simulink model "servomotor_posicao_EKF_Com_Ruido_Posicao"  (R2024b)
settings: Solver=FixedStepAuto  StartTime=0.0  StopTime=tf  FixedStep=1e-6  RelTol=1e-3
values from neighbouring files (symbols this model uses):
  controlador =     [controlador.mat]    (also in projetarControladorPosicaoOtimizacao.m = projetarControladorPosicaoAnalitico(requisitos, planta))
  planta =     [controlador.mat]    (also in kalman.m = obterPlantaServoPosicao())
undefined symbols (not defined in the file or in its folder): Continuous, Time
libraries: ctrlSharedLib x1
settings Model: Creator=mmaximo  LastModifiedBy=phdfo
settings SolverCC: AlgebraicLoopSolver=TrustRegion
settings DebuggingCC: UnconnectedInputMsg=warning  UnconnectedOutputMsg=warning  UnconnectedLineMsg=warning
settings ModelReferenceCC: EnableRefExpFcnMdlSchedulingChecks=on
settings RTWCC: GPUComputeCapability=3.5

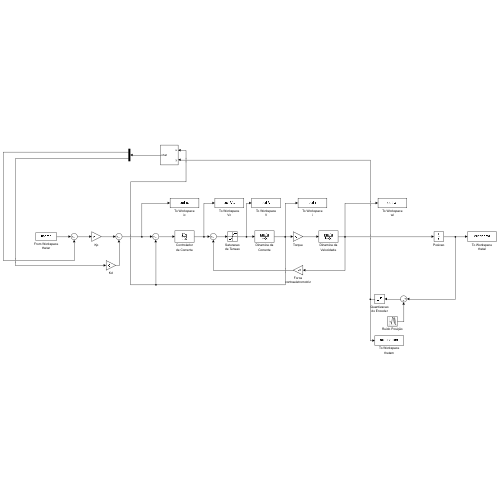
[thumbnail: Simulink's stored preview of the top-level diagram]
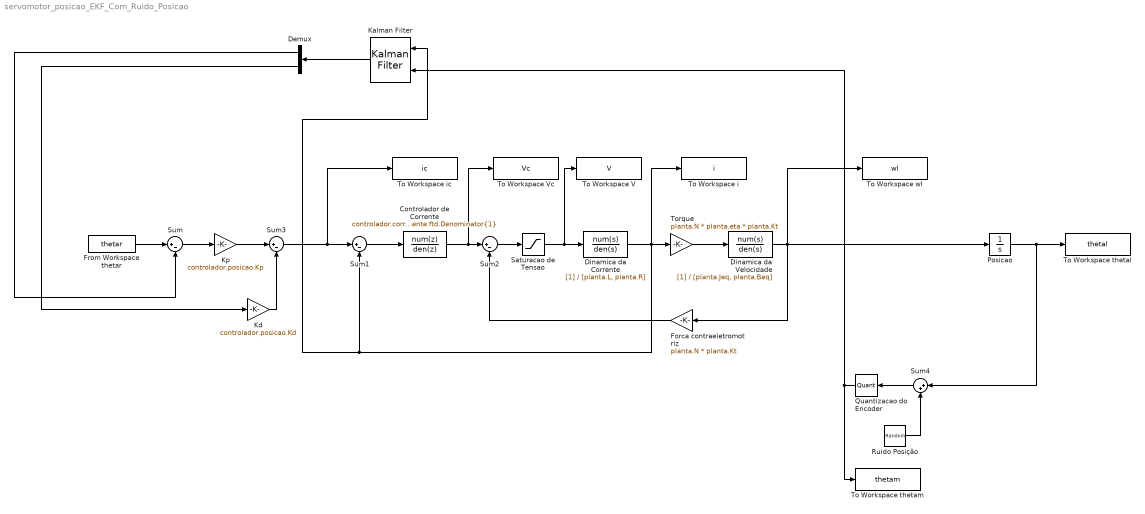
== system servomotor_posicao_EKF_Com_Ruido_Posicao ==
  Controlador de Corrente : DiscreteTransferFcn  Numerator=controlador.corrente.ftd.Numerator{1}  Denominator=controlador.corrente.ftd.Denominator{1}  SampleTime=controlador.corrente.T
  Demux : Demux  Outputs=2
  Dinamica da Corrente : TransferFcn  Denominator=[planta.L, planta.R]
  Dinamica da Velocidade : TransferFcn  Denominator=[planta.Jeq, planta.Beq]
  Forca contraeletromotriz : Gain  Gain=planta.N * planta.Kt
  From Workspace thetar : FromWorkspace  VariableName=thetar
  Kalman Filter : ctrlSharedLib/Kalman Filter  TimeDomain=Continuous-Time  UseCurrentEstimator=on  ModelSource=Individual A, B, C, D matrices  ModelSourceVariable=ss(0.95,1,1,0,1)  A=planta.Kalman.A  B=planta.Kalman.B  C=planta.Kalman.C  D=planta.Kalman.D  NumberOfStates=1  NumberOfInputs=1  NumberOfOutputs=1  InitialEstimateSource=Dialog  X0=0  P0=10  UseK=off  UseGH=off  NumberOfProcessNoiseInputs=1  G=1  TimeInvariantG=on  H=0  TimeInvariantH=on  Q=0.05  TimeInvariantQ=on  R=1  TimeInvariantR=on  N=0  TimeInvariantN=on  AddInputPort=on  AddEnablePort=off  OutputEstimatedY=off  OutputP=off  Ts=-1
  Kd : Gain  Gain=controlador.posicao.Kd
  Kp : Gain  Gain=controlador.posicao.Kp
  Posicao : Integrator
  Quantizacao do Encoder : Quantizer  QuantizationInterval=planta.quantizacaoEncoder
  Ruido Posição : RandomNumber  Tag=Ruido_posicao  Description=Ruido_posicao  SampleTime=0.01
  Saturacao de Tensao : Saturate  UpperLimit=planta.Vmax  LowerLimit=-planta.Vmax
  Sum{,1..3} (4 alike) : Sum  Inputs=|+-
  Sum4 : Sum  Inputs=|++
  To Workspace V : ToWorkspace  VariableName=V  SaveFormat=Structure With Time  SampleTime=1e-6
  To Workspace Vc : ToWorkspace  VariableName=Vc  SaveFormat=Structure With Time  SampleTime=1e-6
  To Workspace i : ToWorkspace  VariableName=i  SaveFormat=Structure With Time  SampleTime=1e-6
  To Workspace ic : ToWorkspace  VariableName=ic  SaveFormat=Structure With Time  SampleTime=1e-6
  To Workspace thetal : ToWorkspace  VariableName=thetal  SaveFormat=Structure With Time  SampleTime=-1
  To Workspace thetam : ToWorkspace  VariableName=thetam  SaveFormat=Structure With Time  SampleTime=-1
  To Workspace wl : ToWorkspace  VariableName=wl  SaveFormat=Structure With Time  SampleTime=1e-6
  Torque : Gain  Gain=planta.N * planta.eta * planta.Kt
  wires:
  From Workspace thetar/1 -> Sum/1
  Dinamica da Velocidade/1 -> To Workspace wl/1, Forca contraeletromotriz/1, Posicao/1
  Torque/1 -> Dinamica da Velocidade/1
  Forca contraeletromotriz/1 -> Sum2/2
  Sum1/1 -> Controlador de Corrente/1
  Sum/1 -> Kp/1
  Posicao/1 -> Sum4/1, To Workspace thetal/1
  Quantizacao do Encoder/1 -> To Workspace thetam/1, Kalman Filter/2
  Kp/1 -> Sum3/1
  Sum3/1 -> To Workspace ic/1, Sum1/1
  Demux/1 -> Sum/2
  Kalman Filter/1 -> Demux/1
  Ruido Posição/1 -> Sum4/2
  Saturacao de Tensao/1 -> To Workspace V/1, Dinamica da Corrente/1
  Sum2/1 -> Saturacao de Tensao/1
  Controlador de Corrente/1 -> To Workspace Vc/1, Sum2/1
  Demux/2 -> Kd/1
  Kd/1 -> Sum3/2
  Sum4/1 -> Quantizacao do Encoder/1
  Dinamica da Corrente/1 -> Kalman Filter/1, Sum1/2, To Workspace i/1, Torque/1
